simulink model "xpcrs232"  (Simulink 5.0)
settings: Solver=FixedStepDiscrete  StartTime=0.0  StopTime=300  RelTol=1e-3
libraries: xpclib x5
settings Model: Creator=mvetsch  LastModifiedBy=ekbas  ExtModeMexFile=ext_xpc  ExtModeTrigMode=oneshot  ExtModeArmWhenConnect=off  SimulationMode=external  LimitDataPoints=off  BlockReductionOpt=off  BooleanDataType=off  RTWSystemTargetFile=xpctarget.tlc  RTWTemplateMakefile=xpc_default_tmf  RTWOptions="-aRollThreshold=5 -aShowEliminatedStatements=1 -aRTWVerbose=1 -aInlineInvariantSignals=0 -aLocalBlockOutputs=0 -aRL32ModeModifier=\"Real-Time\" -aRL32LogTETModifier=1 -aRL32ScopeModifier=1 -aRL32LogBufSizeModifier=100000 -aRL32IRQSourceModifier=\"Timer\" -aRL32ObjectName=\"tg\" -aInlineParameters=0"

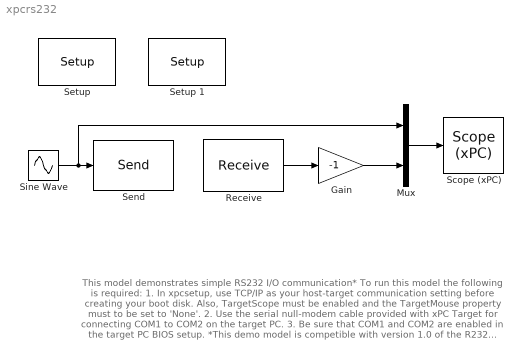
== system xpcrs232 ==
  note: This model demonstrates simple RS232 I/O communication*
      |
      | To run this model the following is required:
      |
      | 1. In xpcsetup, use TCP/IP as your host-target communication setting before creating your boot disk.
      | Also, TargetScope must be enabled and the TargetMouse property must to be set to 'None'.
      |
      | 2. Use the serial null-modem cable provided with xPC Target for connecting COM1 to
      | COM2 on the target PC.
      |
      | 3. Be sure that COM1 and COM2 are enabled in the target PC BIOS setup.
      |
      | *This demo model is competible with version 1.0 of the R232 blocks. Please also see xPCRS232V2
  Gain : Gain  Gain=-1  SaturateOnIntegerOverflow=on
  Mux : Mux  Inputs=2
  "Receive " : xpclib/RS232/Asynchronous Mode/Receive   port=COM2  formatrec='start,%f,stop;'  numb=1  ts=0.01
  "Scope (xPC) " : xpclib/Misc./Scope (xPC)   scopeno=1  scopetype=Target  viewmode=Graphical rolling  grid=on  ylimits=[0,0]  autostart=on  nosamples=250  noprepostsamples=0  interleave=1  triggermode=FreeRun  triggersignal=1  triggerlevel=0.0  triggerslope=either  triggerscope=1  triggersample=0
  "Send " : xpclib/RS232/Asynchronous Mode/Send   port=COM1  formatsend='start,%f,stop;'  wait=off  ts=0.01
  "Setup " : xpclib/RS232/Setup   port=COM1  baudrate=115200  databit=8  stopbit=1  parity=None  protocol=None  sendbuf=1024  recbuf=1024
  Setup 1 : xpclib/RS232/Setup   port=COM2  baudrate=115200  databit=8  stopbit=1  parity=None  protocol=None  sendbuf=1024  recbuf=1024
  Sine Wave : Sin  Frequency=5  SampleTime=0
  wires:
  Sine Wave/1 -> "Send "/1, Mux/1
  "Receive "/1 -> Gain/1
  Gain/1 -> Mux/2
  Mux/1 -> "Scope (xPC) "/1
